simulink model "SingleTrackCANoe"  (R2021b)
settings: Solver=ode1  StartTime=0  StopTime=2  FixedStep=1.0000000000000000e-003  RelTol=1e-3
InitFcn:
  | sampleTime = str2double(get_param(bdroot, 'FixedStep'));
undefined symbols (not defined in the file or in its folder): AccPedalPos, BrakePedalPos, BrakeSwitch, DiscIntNeverNeededParam, DYNA4, EngSpd, IgnitionSwitch, InitialGear, InitialSpeed, IntendedEngTrq, LeftIndicator, MainBrakePress, MaxGear, MDL, MinGear, RefAcc, RefLane, RefLatPos, RefPath, RefPathCurv, RefSpd, RefSpdPreview, RefSpdRetrospect, RightIndicator, SteeringWheelAng, SteeringWheelTrq, UserDefinedRefValue, vm_const
libraries: UtilitiesLibrary x62, simulink x18, WheelSystemModules x14, LongitudinalControllerModules x13, LateralControllerModules x7, AnimationBusselectorModules x5, EnvironmentModules x5, BasicEngineControlModules x5, MiscellaneousControlModules x5, Animation3Modules x4, AuxiliariesModules x4, ReducedTireModules x4
(part 26 of 34)

== system SingleTrackCANoe/SimulationModel/VehicleControl/LateralControl/Enabled LateralControl/ControlSystems ==
  note: How to add user-defined lateral additional inputs to the model:
      |
      | 1. Open the block "LateralControlOutput" by double-clicking on it.
      | 2. Edit the signals "UserDefined.<signalname>" inside by renaming them and setting the unit. You can also add signals to the existing ones.
      | Be careful to always use the prefix "UserDefined." for additional signals!!!
      | 3. Adjust the size of the demux-block of the user-defined signals on the left of the bus-creator so that all ports can be connected.
      | 4. Save the model to apply your changes.
  Phase[-] : Inport
  TaskIdentifiers : Inport  Port=2
  SourceIdentifiers : Inport  Port=3
  ControlInputs : Inport  Port=4
  UserDefinedSignals : Inport  Port=5
  VehicleInfo : Inport  Port=6
  CtrlSystemsAbscissae : Inport  Port=7
  Bus Selector1 : BusSelector  OutputSignals=SteeringWheelTrq[Nm],SteeringWheelInputSwitch[-]
  Bus Selector2 : BusSelector  OutputSignals=LeftIndicator,RightIndicator
  Control Systems Parameters : Subsystem
  Demux : Demux  Outputs=2
  DynaSystemInfo : Subsystem  Tag=DynaSystemInfo
      mask init:
      | data = get_param(gcb, 'UserData');
      settings: OpenFcn=DYNA4.ModelHandling.System.ShowEditSystemInformationDialog(gcb);
      mask Display: disp(['Type = ', data.type, '\nName = ', data.name ])
  Lateral Controller : Subsystem
  LateralControlOutput : Subsystem  Tag=TESIS DYNAware Interface Block  mask{NeedsUpdate=off, SignalInfo=|}
      mask SignalInfo=|
      | {
      |   "Version": "4.6",
      |   "MuxedOutputBusName": "LateralControl",
      |   "MuxedInputBusName": "fromCTRL",
      |   "MuxedInputSelected": false,
      |   "MuxedOutputSelected": true,
      |   "SignalData": [
      |     {
      |       "initialValue": "0.0",
      |       "name": "SteeringWheelAng[rad]",
      |       "comment": "Steering wheel angle",
      |       "minString": "",
      |       "maxString": "",
      |       "width": 1,
      |       "dataType": 0,
      |       "signalType": 0,
      |       "createSignal": false,
      |       "outputName": "SteeringWheelAng[rad]",
      |       "generateSignalAccessBlock": false,
      |       "accessId": "$(parentId).$(blockName).$(outputName)"
      |     },
      |     {
      |       "initialValue": "0.0",
      |       "name": "SteeringWheelTrq[Nm]",
      |       "comment": "Steering wheel torque",
      |       "minString": "",
      |       "maxString": "",
      |       "width": 1,
      |       "dataType": 0,
      |       "signalType": 0,
      |       "createSignal": false,
      |       "outputName": "SteeringWheelTrq[Nm]",
      |       "generateSignalAccessBlock": false,
      |       "accessId": "$(parentId).$(blockName).$(outputName)"
      |     },
      |     {
      |       "initialValue": "0.0",
      |       "name": "SteeringWheelInputSwitch[-]",
      |       "comment": "Steering wheel input switch (0: angle, 1: torque)",
      |       "minString": "",
      |       "maxString": "",
      |       "width": 1,
      |       "dataType": 0,
      |       "signalType": 0,
      |       "createSignal": false,
      |       "outputName": "SteeringWheelInputSwitch[-]",
      |       "generateSignalAccessBlock": false,
      |       "accessId": "$(parentId).$(blockName).$(outputName)"
      |     },
      |     {
      |       "initialValue": "0.0",
      |       "name": "UserDefinedRefValue[-]",
      |       "comment": "User-defined reference value",
      |       "minString": "",
      |       "maxString": "",
      |       "width": 1,
      |       "dataType": 0,
      |       "signalType": 0,
      |       "createSignal": false,
      |       "outputName": "UserDefinedRefValue[-]",
      |       "generateSignalAccessBlock": false,
      |       "accessId": "$(parentId).$(blockName).$(outputName)"
      |     },
      |     {
      |       "initialValue": "0.0",
      |       "name": "LeftIndicator[0;1]",
      |       "comment": "Left indicator state",
      |       "minString": "",
      |       "maxString": "",
      |       "width": 1,
      |       "dataType": 0,
      |       "signalType": 0,
      |       "createSignal": false,
      |       "outputName": "LeftIndicator[0;1]",
      |       "generateSignalAccessBlock": false,
      |       "accessId": "$(parentId).$(blockName).$(outputName)"
      |     },
      |     {
      |       "initialValue": "0.0",
      |       "name": "RightIndicator[0;1]",
      |       "comment": "Right indicator state",
      |       "minString": "",
      |       "maxString": "",
      |       "width": 1,
      |       "dataType": 0,
      |       "signalType": 0,
      |       "createSignal": false,
      |       "outputName": "RightIndicator[0;1]",
      |       "generateSignalAccessBlock": false,
      |       "accessId": "$(parentId).$(blockName).$(outputName)"
      |     },
      |     {
      |       "initialValue": "0.0",
      |       "name": "LateralPhase[-]",
      |       "comment": "Lateral phase number",
      |       "minString": "",
      |       "maxString": "",
      |       "width": 1,
      |       "dataType": 0,
      |       "signalType": 0,
      |       "createSignal": false,
      |       "outputName": "LateralPhase[-]",
      |       "generateSignalAccessBlock": false,
      |       "accessId": "$(parentId).$(blockName).$(outputName)"
      |     },
      |     {
      |       "initialValue": "0.0",
      |       "name": "UserDefined.UserDefined1[-]",
      |       "comment": "User-defined additional input 1 (can be edited by the user)",
      |       "minString": "",
      |       "maxString": "",
      |       "width": 1,
      |       "dataType": 0,
      |       "signalType": 0,
      |       "createSignal": false,
      |       "outputName": "UserDefined1[-]",
      |       "generateSignalAccessBlock": false,
      |       "accessId": "$(parentId).$(blockName).$(outputName)"
      |     },
      |     {
      |       "initialValue": "0.0",
      |       "name": "UserDefined.UserDefined2[-]",
      |       "comment": "User-defined additional input 2 (can be edited by the user)",
      |       "minString": "",
      |       "maxString": "",
      |       "width": 1,
      |       "dataType": 0,
      |       "signalType": 0,
      |       "createSignal": false,
      |       "outputName": "UserDefined2[-]",
      |       "generateSignalAccessBlock": false,
      |       "accessId": "$(parentId).$(blockName).$(outputName)"
      |     }
      |   ]
      | }
      mask prompts: NeedsUpdate "Specify, if subsystem content needs to be updated"; SignalInfo "Signal Info (json)"
      mask help: DYNA4 Interface Block Version 4.6
      mask init:
      | blockName = get_param(gcbh, 'Name');
      | parentId = DYNA4.ModelHandling.AccessID.getFromHierarchy(gcbh);
      | TD.InterfaceBlock.ModelCallbacks.GenerateContent(gcb);
      settings: DeleteFcn=TD.InterfaceBlock.ModelCallbacks.CloseGUI( gcbh );  NameChangeFcn=TD.InterfaceBlock.ModelCallbacks.BlockRenamedHandler(gcbh);  OpenFcn=TD.InterfaceBlock.ModelCallbacks.OpenGUI( gcbh );  CloseFcn=TD.InterfaceBlock.ModelCallbacks.CloseGUI( gcbh );
      mask Display:
      | image('InterfaceBlock.png','center');
      | port_label('input',1, 'SteeringWheelAng[rad]');
      | port_label('input',2, 'SteeringWheelTrq[Nm]');
      | port_label('input',3, 'SteeringWheelInputSwitch[-]');
      | port_label('input',4, 'UserDefinedRefValue[-]');
      | port_label('input',5, 'LeftIndicator[0;1]');
      | port_label('input',6, 'RightIndicator[0;1]');
      | port_label('input',7, 'LateralPhase[-]');
      | port_label('input',8, 'UserDefined.UserDefined1[-]');
      | port_label('input',9, 'UserDefined.UserDefined2[-]');
      | port_label('output',1, 'LateralControl');
  SteeringWheelLimitation : Subsystem
  LateralControl : Outport  VectorParamsAs1DForOutWhenUnconnected=off
  ControllerParameters : Outport  Port=2  VectorParamsAs1DForOutWhenUnconnected=off
  wires:
  LateralControlOutput/1(LateralControl___UNIQUE_1) -> LateralControl/1
  SourceIdentifiers/1 -> Lateral Controller/2(SourceIdentifiers)
  VehicleInfo/1 -> Lateral Controller/5(VehicleInfo)
  Bus Selector2/1 -> LateralControlOutput/5(LeftIndicator[0;1]___UNIQUE_1)  "<LeftIndicator>"
  TaskIdentifiers/1 -> Control Systems Parameters/1(TaskIdentifier), Lateral Controller/1(TaskIdentifiers)
  Lateral Controller/2(UserDefinedRefValue[-]) -> LateralControlOutput/4(UserDefinedRefValue[-]___UNIQUE_1)
  Bus Selector2/2 -> LateralControlOutput/6(RightIndicator[0;1]___UNIQUE_1)  "<RightIndicator>"
  Lateral Controller/1(SteeringWheelDemands) -> Bus Selector1/1, SteeringWheelLimitation/1(SteeringWheelDemands)
  ControlInputs/1 -> Bus Selector2/1, SteeringWheelLimitation/2(ControlInputs), Lateral Controller/3(ControlInputs)
  SteeringWheelLimitation/1(ModifiedSteeringWhlAng[rad]) -> LateralControlOutput/1(SteeringWheelAng[rad]___UNIQUE_1)
  CtrlSystemsAbscissae/1 -> Control Systems Parameters/2(CtrlSystemsAbscissae)
  Demux/1 -> LateralControlOutput/8(UserDefined1[-]___UNIQUE_1)
  Demux/2 -> LateralControlOutput/9(UserDefined2[-]___UNIQUE_1)
  Control Systems Parameters/1(ControllerParameters) -> Lateral Controller/4(ControllerParameters), ControllerParameters/1
  UserDefinedSignals/1 -> Demux/1
  Bus Selector1/2 -> LateralControlOutput/3(SteeringWheelInputSwitch[-]___UNIQUE_1)  "<SteeringWheelInputSwitch[-]>"
  Bus Selector1/1 -> LateralControlOutput/2(SteeringWheelTrq[Nm]___UNIQUE_1)  "<SteeringWheelTrq[Nm]>"
  Phase[-]/1 -> LateralControlOutput/7(LateralPhase[-]___UNIQUE_1)

== system SingleTrackCANoe/SimulationModel/VehicleControl/LateralControl/Enabled LateralControl/ControlSystemsPreprocessor ==
  SchedulerAbscissae : Inport
  PhaseTerminationVals : Inport  Port=2
  LatCTRL : Inport  Port=3
  ExtCtrlVariablesEnforced : Inport  Port=4
  ExtCtrlVals : Inport  Port=5
  ControllerParameters : Inport  Port=6
  VehicleInfo : Inport  Port=7
  "External Presetting of Controller " : Subsystem
  Generation of Guidance Data : Subsystem
  Generation of Hold Data : Subsystem
  Maneuver : ManeuverControlModules/LateralManeuver  DATA_NODE=MDL.VehicleControl.LateralControl.Maneuver  Scheduler=MDL.VehicleControl.LateralControl.Maneuver.Scheduler
  Switch between Data Sources : Subsystem
  Phase[-] : Outport  VectorParamsAs1DForOutWhenUnconnected=off
  TaskIdentifiers : Outport  Port=2  VectorParamsAs1DForOutWhenUnconnected=off
  SourceIdentifiers : Outport  Port=3  VectorParamsAs1DForOutWhenUnconnected=off
  ControlInputs : Outport  Port=4  VectorParamsAs1DForOutWhenUnconnected=off
  UserDefinedSignals : Outport  Port=5  VectorParamsAs1DForOutWhenUnconnected=off
  wires:
  ExtCtrlVals/1 -> Switch between Data Sources/4(ExternalData)
  Generation of Hold Data/1(HoldData) -> Switch between Data Sources/3(HoldData)
  Maneuver/5 -> Switch between Data Sources/2(ControlInputs)
  ControllerParameters/1 -> Generation of Guidance Data/3(ControllerParameters)
  VehicleInfo/1 -> Generation of Hold Data/3(VehicleInfo), Generation of Guidance Data/4(VehicleInfo)
  Maneuver/3 -> "External Presetting of Controller "/1(TaskIdentifiers)
  Maneuver/4 -> "External Presetting of Controller "/2(SourceIdentifiers)
  Maneuver/2 -> Generation of Hold Data/1(PhaseTrigger)
  PhaseTerminationVals/1 -> Maneuver/2
  SchedulerAbscissae/1 -> Maneuver/1
  ExtCtrlVariablesEnforced/1 -> "External Presetting of Controller "/3(ExtCtrlVariablesEnforced)
  "External Presetting of Controller "/1(ModifiedTaskIdentifiers) -> TaskIdentifiers/1, Generation of Guidance Data/1(TaskIdentifiers)
  "External Presetting of Controller "/2(ModifiedSourceIdentifiers) -> SourceIdentifiers/1, Switch between Data Sources/1(SourceIdentifiers)
  Generation of Guidance Data/1(ExtendedControlInputs) -> ControlInputs/1
  Switch between Data Sources/1(SwitchedControlInputs) -> Generation of Guidance Data/2(ControlInputs)
  LatCTRL/1 -> Generation of Hold Data/2(LatCTRL)
  Maneuver/6 -> UserDefinedSignals/1
  Maneuver/1 -> Phase[-]/1

== system SingleTrackCANoe/SimulationModel/VehicleControl/LateralControl/Enabled LateralControl/DynaSystemInfo ==

== system SingleTrackCANoe/SimulationModel/VehicleControl/LongitudinalControl/ControlSystems/Brake System Switch and Pedal Limitation ==
  note: SUBTASK_LONG_ACC_BRAKEPEDAL = 1;
      | 	SUBTASK_LONG_ACC_BRAKEPRESSURE_MAIN = 2;
      | 	SUBTASK_LONG_ACC_BRAKEPRESSURES = 3;
  note: TASK_LONG_ACC_BRAKE_INPUTS = 1;
      | 	TASK_LONG_SPEED_CONTROL = 2;
      | 	TASK_LONG_ACCELERATION_CONTROL = 3;
      | 	TASK_LONG_USER_DEFINED = 4;
  ControlOutputs : Inport
  TaskIdentifiers : Inport  Port=2
  VehicleInfoSpeedControl : Inport  Port=3
  ControlInputs : Inport  Port=4
  AccBrakeLimitation : Subsystem
  BrakeSwitch = 1 : Subsystem  TreatAsAtomicUnit=on
  BrakeSwitch = 2 : Subsystem  TreatAsAtomicUnit=on
  Bus Assignment : BusAssignment  AssignedSignals=BrakeSwitch,AccPedalPos,BrakePedalPos,MainBrakePress
  Bus Selector : BusSelector  OutputSignals=VehicleDriverInfo_MaxMainBrakePress[Pa]
  Bus Selector1 : BusSelector  OutputSignals=AccPedalPos,BrakePedalPos,MainBrakePress
  Bus Selector2 : BusSelector  OutputSignals=BrakePedalPos,MainBrakePressure
  Bus Selector4 : BusSelector  OutputSignals=FrontLeftWheelBrakePress,FrontRightWheelBrakePress,RearLeftWheelBrakePress,RearRightWheelBrakePress,Rear2LeftWheelBrakePress,Rear2RightWheelBrakePress,Rear3LeftWheelBrakePress,Rear3RightWheelBrakePress,TrailerFrontLeftWheelBrakePress,TrailerFrontRightWheelBrakePress,TrailerRearLeftWheelBrakePress,TrailerRearRightWheelBrakePress,TrailerRear2LeftWheelBrakePress,TrailerRear2RightWheelBrakePress,TrailerRear3LeftWheelBrakePress,TrailerRear3RightWheelBrakePress  OutputAsBus=on
  Bus Selector7 : BusSelector  OutputSignals=Task,Subtask
  Constant : Constant  Value=vm_const('SUBTASK_LONG_ACC_BRAKEPEDAL')
  "Constant, Table, Automatic, Sine4" : simulink/Logic and Bit Operations/Compare To Constant  relop=~=  const=vm_const('TASK_LONG_ACC_BRAKE_INPUTS')  OutDataTypeStr=uint8  ZeroCross=off
  Default : Subsystem  TreatAsAtomicUnit=on
  Merge : Merge  Inputs=3
  Switch : Switch  Criteria=u2 > Threshold
  Switch Case : SwitchCase  CaseConditions={1, 2}
  ModifiedControlOutputs : Outport  VectorParamsAs1DForOutWhenUnconnected=off
  wires:
  Bus Selector1/1 -> AccBrakeLimitation/1(AccPedalPos[0_1])  "<AccPedalPos>"
  AccBrakeLimitation/2(BrakePedalPosLimited) -> Bus Assignment/4
  AccBrakeLimitation/1(AccPedalPosLimited) -> Bus Assignment/3
  Bus Selector2/1 -> AccBrakeLimitation/2(BrakePedalPos[0_1])  "<BrakePedalPos>"
  Bus Selector2/2 -> Bus Assignment/5  "<MainBrakePressure>"
  ControlInputs/1 -> AccBrakeLimitation/3(ControlInputs)
  Default/1(BrakeOutput) -> Merge/3
  BrakeSwitch = 2/1(BrakeOutput) -> Merge/2
  BrakeSwitch = 1/1(BrakeOutput) -> Merge/1
  Bus Selector1/3 -> BrakeSwitch = 2/1(MainBrakePressure)  "<MainBrakePress>"
  Bus Selector4/1 -> Default/1(WheelBrakePressures), BrakeSwitch = 1/2(WheelBrakePressures)
  Bus Selector/1 -> Default/2(MaxMainBrakePressure), BrakeSwitch = 2/2(MaxMainBrakePressure)  "<VehicleDriverInfo_MaxMainBrakePress[Pa]>"
  Bus Assignment/1 -> ModifiedControlOutputs/1
  Bus Selector1/2 -> BrakeSwitch = 1/1(BrakePedalPos)  "<BrakePedalPos>"
  Merge/1 -> Bus Selector2/1
  Switch Case/3 -> Default/Action
  Switch Case/2 -> BrakeSwitch = 2/Action
  Switch Case/1 -> BrakeSwitch = 1/Action
  TaskIdentifiers/1 -> Bus Selector7/1
  Bus Selector7/1 -> "Constant, Table, Automatic, Sine4"/1  "<Task>"
  "Constant, Table, Automatic, Sine4"/1 -> Switch/2
  Constant/1 -> Switch/1
  Bus Selector7/2 -> Switch/3  "<Subtask>"
  Switch/1 -> Bus Assignment/2, Switch Case/1  "BrakeSwitch[-]"
  VehicleInfoSpeedControl/1 -> Bus Selector/1
  ControlOutputs/1 -> Bus Assignment/1, Bus Selector1/1, Bus Selector4/1
